simulink model "Closed_Loop_LEDControllers"  (R2024b)
settings: configuration reference "ConfigSet_Sim_ASW" (kept outside this file)
model workspace (MAT data in the model file):
  TsModel = 0.001
libraries: SEPIC_utilities x6
settings Model: DataDictionary=LocalDataD_Closed_Loop_LEDControllers.sldd  ExtModeTrigDuration=8  Creator=vivekr  LastModifiedBy=vlenzi
settings ConfigSetRef: SourceName=ConfigSet_Sim_ASW

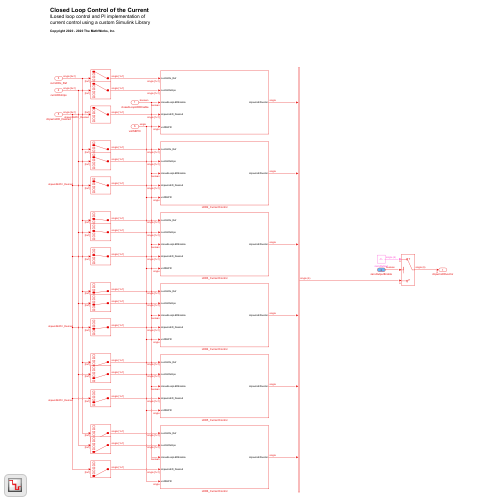
[thumbnail: Simulink's stored preview of the top-level diagram]
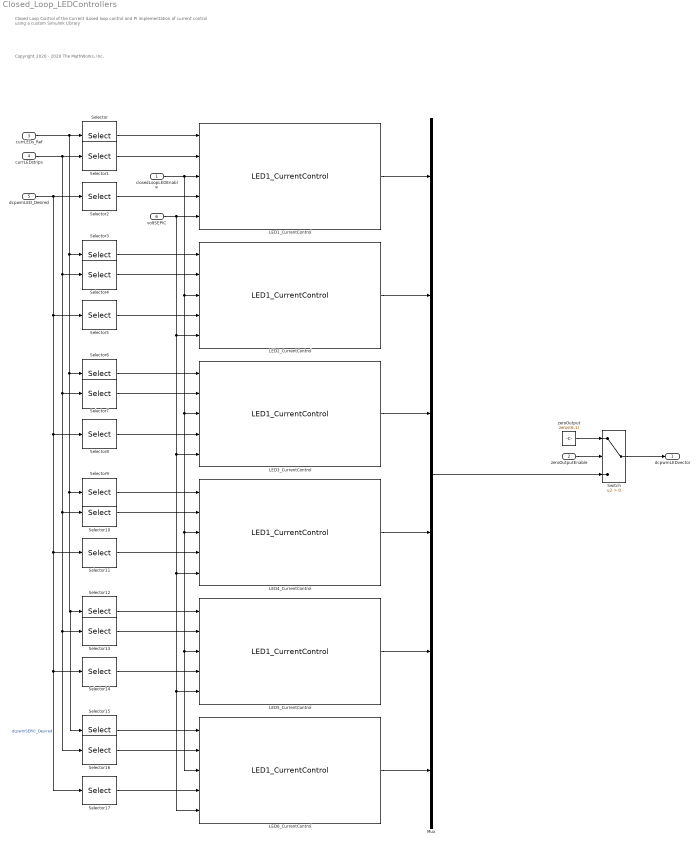
== system Closed_Loop_LEDControllers ==
  note: Closed Loop Control of the Current
      | lLosed loop control and PI implementation of current control using a custom Simulink Library
  note: Copyright 2020 - 2020 The MathWorks, Inc.
  closedLoopLEDEnable : Inport  Unit=1  SampleTime=TsModel
  zeroOutputEnable : Inport  Port=2  OutDataTypeStr=boolean  Unit=1  PortDimensions=1  SampleTime=TsModel
  currLEDs_Ref : Inport  Port=3  OutDataTypeStr=single  Unit=mA  PortDimensions=[6 1]  SampleTime=TsModel
  currLEDstrips : Inport  Port=4  OutDataTypeStr=single  Unit=mA  PortDimensions=[6 1]  SampleTime=TsModel
  dcpwmLED_Desired : Inport  Port=5  OutDataTypeStr=single  Unit=1  PortDimensions=[6 1]  SampleTime=TsModel
  voltSEPIC : Inport  Port=6  OutDataTypeStr=single  Unit=V  PortDimensions=1  SampleTime=TsModel
  LED1_CurrentControl : SEPIC_utilities/LED1_CurrentControl  PGain=CurrCtrlr_PGain  IGain=CurrCtrlr_IGain
  LED2_CurrentControl : SEPIC_utilities/LED1_CurrentControl  PGain=CurrCtrlr_PGain  IGain=CurrCtrlr_IGain
  LED3_CurrentControl : SEPIC_utilities/LED1_CurrentControl  PGain=CurrCtrlr_PGain  IGain=CurrCtrlr_IGain
  LED4_CurrentControl : SEPIC_utilities/LED1_CurrentControl  PGain=CurrCtrlr_PGain  IGain=CurrCtrlr_IGain
  LED5_CurrentControl : SEPIC_utilities/LED1_CurrentControl  PGain=CurrCtrlr_PGain  IGain=CurrCtrlr_IGain
  LED6_CurrentControl : SEPIC_utilities/LED1_CurrentControl  PGain=CurrCtrlr_PGain  IGain=CurrCtrlr_IGain
  Mux : Mux  Inputs=6
  Selector : Selector  InputPortWidth=6  IndexOptions=Index vector (dialog)  Indices=1  OutputSizes=1
  Selector1 : Selector  InputPortWidth=6  IndexOptions=Index vector (dialog)  Indices=1  OutputSizes=1
  Selector10 : Selector  InputPortWidth=6  IndexOptions=Index vector (dialog)  Indices=4  OutputSizes=1
  Selector11 : Selector  InputPortWidth=6  IndexOptions=Index vector (dialog)  Indices=4  OutputSizes=1
  Selector12 : Selector  InputPortWidth=6  IndexOptions=Index vector (dialog)  Indices=5  OutputSizes=1
  Selector13 : Selector  InputPortWidth=6  IndexOptions=Index vector (dialog)  Indices=5  OutputSizes=1
  Selector14 : Selector  InputPortWidth=6  IndexOptions=Index vector (dialog)  Indices=5  OutputSizes=1
  Selector15 : Selector  InputPortWidth=6  IndexOptions=Index vector (dialog)  Indices=6  OutputSizes=1
  Selector16 : Selector  InputPortWidth=6  IndexOptions=Index vector (dialog)  Indices=6  OutputSizes=1
  Selector17 : Selector  InputPortWidth=6  IndexOptions=Index vector (dialog)  Indices=6  OutputSizes=1
  Selector2 : Selector  InputPortWidth=6  IndexOptions=Index vector (dialog)  Indices=1  OutputSizes=1
  Selector3 : Selector  InputPortWidth=6  IndexOptions=Index vector (dialog)  Indices=2  OutputSizes=1
  Selector4 : Selector  InputPortWidth=6  IndexOptions=Index vector (dialog)  Indices=2  OutputSizes=1
  Selector5 : Selector  InputPortWidth=6  IndexOptions=Index vector (dialog)  Indices=2  OutputSizes=1
  Selector6 : Selector  InputPortWidth=6  IndexOptions=Index vector (dialog)  Indices=3  OutputSizes=1
  Selector7 : Selector  InputPortWidth=6  IndexOptions=Index vector (dialog)  Indices=3  OutputSizes=1
  Selector8 : Selector  InputPortWidth=6  IndexOptions=Index vector (dialog)  Indices=3  OutputSizes=1
  Selector9 : Selector  InputPortWidth=6  IndexOptions=Index vector (dialog)  Indices=4  OutputSizes=1
  Switch : Switch  Criteria=u2 > Threshold  SaturateOnIntegerOverflow=off  InputSameDT=off
  zeroOutput : Constant  Value=zeros(6,1)  OutDataTypeStr=single
  dcpwmLEDvector : Outport  Unit=1  SampleTime=TsModel  VectorParamsAs1DForOutWhenUnconnected=off
  wires:
  Selector/1 -> LED1_CurrentControl/1
  Selector1/1 -> LED1_CurrentControl/2
  Selector2/1 -> LED1_CurrentControl/4
  LED1_CurrentControl/1 -> Mux/1
  Mux/1 -> Switch/3
  LED2_CurrentControl/1 -> Mux/2
  Selector3/1 -> LED2_CurrentControl/1
  Selector4/1 -> LED2_CurrentControl/2
  Selector5/1 -> LED2_CurrentControl/4
  Selector8/1 -> LED3_CurrentControl/4
  Selector7/1 -> LED3_CurrentControl/2
  Selector6/1 -> LED3_CurrentControl/1
  LED3_CurrentControl/1 -> Mux/3
  LED5_CurrentControl/1 -> Mux/5
  Selector12/1 -> LED5_CurrentControl/1
  Selector13/1 -> LED5_CurrentControl/2
  Selector14/1 -> LED5_CurrentControl/4
  Selector11/1 -> LED4_CurrentControl/4
  Selector10/1 -> LED4_CurrentControl/2
  Selector9/1 -> LED4_CurrentControl/1
  LED4_CurrentControl/1 -> Mux/4
  Selector17/1 -> LED6_CurrentControl/4
  Selector16/1 -> LED6_CurrentControl/2
  Selector15/1 -> LED6_CurrentControl/1
  voltSEPIC/1 -> LED1_CurrentControl/5, LED2_CurrentControl/5, LED3_CurrentControl/5, LED4_CurrentControl/5, LED6_CurrentControl/5, LED5_CurrentControl/5
  dcpwmLED_Desired/1 -> Selector11/1, Selector17/1, Selector14/1, Selector8/1, Selector5/1, Selector2/1  "dcpwmSEPIC_Desired"
  currLEDstrips/1 -> Selector10/1, Selector16/1, Selector13/1, Selector7/1, Selector4/1, Selector1/1
  closedLoopLEDEnable/1 -> LED1_CurrentControl/3, LED2_CurrentControl/3, LED3_CurrentControl/3, LED4_CurrentControl/3, LED6_CurrentControl/3, LED5_CurrentControl/3
  currLEDs_Ref/1 -> Selector9/1, Selector15/1, Selector12/1, Selector6/1, Selector3/1, Selector/1
  LED6_CurrentControl/1 -> Mux/6
  zeroOutput/1 -> Switch/1
  zeroOutputEnable/1 -> Switch/2
  Switch/1 -> dcpwmLEDvector/1
